simulink model "ES259A_BattVltgCorrln"  (R2013b)
settings: Solver=FixedStepDiscrete  SolverMode=SingleTasking  StartTime=0.0  StopTime=Inf  FixedStep=0.002  RelTol=1e-3
values from neighbouring files (symbols this model uses):
  BattVltgCorrlnAllwdVltgDif = DataDict.Calibration    [ES259A_BattVltgCorrln_DataDict.m]
  BattVltgCorrlnBattLoVltg = DataDict.Calibration    [ES259A_BattVltgCorrln_DataDict.m]
  BattVltgCorrlnBattOverVltg = DataDict.Calibration    [ES259A_BattVltgCorrln_DataDict.m]
  BattVltgCorrlnBattUnderVltg = DataDict.Calibration    [ES259A_BattVltgCorrln_DataDict.m]
  BattVltgCorrlnNtc0x03C0x0440x04CFailStep = DataDict.Calibration    [ES259A_BattVltgCorrln_DataDict.m]
  BattVltgCorrlnNtc0x03C0x0440x04CPassStep = DataDict.Calibration    [ES259A_BattVltgCorrln_DataDict.m]
  BattVltgCorrlnNtc0x03DFailStep = DataDict.Calibration    [ES259A_BattVltgCorrln_DataDict.m]
  BattVltgCorrlnNtc0x03DPassStep = DataDict.Calibration    [ES259A_BattVltgCorrln_DataDict.m]
  BattVltgCorrlnNtc0x0B0FailStep = DataDict.Calibration    [ES259A_BattVltgCorrln_DataDict.m]
  BattVltgCorrlnNtc0x0B0PassStep = DataDict.Calibration    [ES259A_BattVltgCorrln_DataDict.m]
  BattVltgCorrlnNtc0x0B1FailStep = DataDict.Calibration    [ES259A_BattVltgCorrln_DataDict.m]
  BattVltgCorrlnNtc0x0B1PassStep = DataDict.Calibration    [ES259A_BattVltgCorrln_DataDict.m]
  BattVltgCorrlnNtc0x0B5FailStep = DataDict.Calibration    [ES259A_BattVltgCorrln_DataDict.m]
  BattVltgCorrlnNtc0x0B5PassStep = DataDict.Calibration    [ES259A_BattVltgCorrln_DataDict.m]
  BattVltgCorrlnRcvrlBattLoVltg = DataDict.Calibration    [ES259A_BattVltgCorrln_DataDict.m]
  BattVltgCorrlnRcvrlBattOverVltg = DataDict.Calibration    [ES259A_BattVltgCorrln_DataDict.m]
  BattVltgCorrlnRcvrlBattUnderVltg = DataDict.Calibration    [ES259A_BattVltgCorrln_DataDict.m]
  BattVltgCorrlnSysMinVltg = DataDict.ImprtdCal    [ES250A_BattVltg_DataDict.m]    (also in ES259A_BattVltgCorrln_DataDict.m = DataDict.Calibration)
  BattVltgSwdMax = DataDict.Calibration    [ES250A_BattVltg_DataDict.m]
  ELECGLBPRM_STRTUPSTPWRDISCNCTBTESTCMPL_CNT_U08 = DataDict.Constant    [ES999A_ElecGlbPrm_DataDict.m]
  SYSVLTGFLTDUALIVTR_CNT_U08 = DataDict.Constant    [ES259A_BattVltgCorrln_DataDict.m]
undefined symbols (not defined in the file or in its folder): NtcNr1, NtcSts1, SigQlfr1
libraries: simulink x14
(part 3 of 7)

== system ES259A_BattVltgCorrln/BattVltgCorrln/BattVltgCorrlnPer1/Battery Voltage Diagnostics/Inhibition Off/BattVltg > OverVltg/SetNtcStsB0 ==
  note: Only pass values 2 or 3 as input to NtcSts.
      | 2: PrePassd
      | 3: PreFaild
  NtcNr : Inport
  NtcStInfo : Inport  Port=2
  NtcSts : Inport  Port=3
  DebStep : Inport  Port=4
  Copyright1 : Subsystem  Description=|  mask(Copyright Information){none=on}
      | Copyright info block.                                               
      |                                                                     
      | Place copyright information at the top of every subsystem in design.
      mask prompts: none "No parameters"
      mask help: Place copyright information at the top of every subsystem in design.
      mask Display:
      | NxtrConf = 'Nexteer Confidential';
      | 
      | sys = bdroot; %handle for the current model ("system")
      | first = get_param(sys,'Created');
      | if(isempty(first))
      |     first = datestr(now,'yyyy');
      | else
      |     first = first(end-3:end);  %year is last four digits
      | end
      | 
      | last = get_param(sys,'LastModifiedDate');
      | if isempty(last)
      |     last = datestr(now,'yyyy');
      | else
      |     last = last(end-3:end);
      | end
      | 
      | if strcmp(first,last)
      |     fprintf('%s\nCopyright  %s Nexteer',NxtrConf,first);
      | else
      |     fprintf('%s\n%s%s-%s Nexteer',NxtrConf,char(169),first,last);
      | end
  Data Store Write1 : DataStoreWrite  RequirementInfo={} %GIDa_a76b7c1b_e703_40d3_920b_5685c046c797  DataStoreName=NtcQlfr44
  ISO Fault Debounce Design NOT TO BE IMPLEMENTED IN THIS FDD USED ONLY FOR SIMULATION PURPOSES : Stateflow chart  TreatAsAtomicUnit=on
  Only here because I could not get model to run with enumerations in the stateflow diagram : DataTypeConversion  OutDataTypeStr=uint8
  Terminator : Terminator
  Terminator1 : Terminator
  wires:
  NtcStInfo/1 -> Terminator1/1
  NtcNr/1 -> Terminator/1
  NtcSts/1 -> Only here because I could not get model to run with enumerations in the stateflow diagram/1
  DebStep/1 -> ISO Fault Debounce Design NOT TO BE IMPLEMENTED IN THIS FDD USED ONLY FOR SIMULATION PURPOSES/2(DebStep)
  Only here because I could not get model to run with enumerations in the stateflow diagram/1 -> ISO Fault Debounce Design NOT TO BE IMPLEMENTED IN THIS FDD USED ONLY FOR SIMULATION PURPOSES/1(NtcSts)
  ISO Fault Debounce Design NOT TO BE IMPLEMENTED IN THIS FDD USED ONLY FOR SIMULATION PURPOSES/1(Qualifier) -> Data Store Write1/1

== system ES259A_BattVltgCorrln/BattVltgCorrln/BattVltgCorrlnPer1/Battery Voltage Diagnostics/Inhibition Off/BattVltg > OverVltg/SetNtcStsB1 ==
  note: Only pass values 2 or 3 as input to NtcSts.
      | 2: PrePassd
      | 3: PreFaild
  NtcNr : Inport
  NtcStInfo : Inport  Port=2
  NtcSts : Inport  Port=3
  DebStep : Inport  Port=4
  Copyright1 : Subsystem  Description=|  mask(Copyright Information){none=on}
      | Copyright info block.                                               
      |                                                                     
      | Place copyright information at the top of every subsystem in design.
      mask prompts: none "No parameters"
      mask help: Place copyright information at the top of every subsystem in design.
      mask Display:
      | NxtrConf = 'Nexteer Confidential';
      | 
      | sys = bdroot; %handle for the current model ("system")
      | first = get_param(sys,'Created');
      | if(isempty(first))
      |     first = datestr(now,'yyyy');
      | else
      |     first = first(end-3:end);  %year is last four digits
      | end
      | 
      | last = get_param(sys,'LastModifiedDate');
      | if isempty(last)
      |     last = datestr(now,'yyyy');
      | else
      |     last = last(end-3:end);
      | end
      | 
      | if strcmp(first,last)
      |     fprintf('%s\nCopyright  %s Nexteer',NxtrConf,first);
      | else
      |     fprintf('%s\n%s%s-%s Nexteer',NxtrConf,char(169),first,last);
      | end
  Data Store Write1 : DataStoreWrite  RequirementInfo={} %GIDa_e78ef1d1_c2fb_41bc_8318_ed3d0db9f38f  DataStoreName=NtcQlfr44
  ISO Fault Debounce Design NOT TO BE IMPLEMENTED IN THIS FDD USED ONLY FOR SIMULATION PURPOSES : Stateflow chart  TreatAsAtomicUnit=on
  Only here because I could not get model to run with enumerations in the stateflow diagram : DataTypeConversion  OutDataTypeStr=uint8
  Terminator : Terminator
  Terminator1 : Terminator
  wires:
  NtcStInfo/1 -> Terminator1/1
  NtcNr/1 -> Terminator/1
  NtcSts/1 -> Only here because I could not get model to run with enumerations in the stateflow diagram/1
  DebStep/1 -> ISO Fault Debounce Design NOT TO BE IMPLEMENTED IN THIS FDD USED ONLY FOR SIMULATION PURPOSES/2(DebStep)
  Only here because I could not get model to run with enumerations in the stateflow diagram/1 -> ISO Fault Debounce Design NOT TO BE IMPLEMENTED IN THIS FDD USED ONLY FOR SIMULATION PURPOSES/1(NtcSts)
  ISO Fault Debounce Design NOT TO BE IMPLEMENTED IN THIS FDD USED ONLY FOR SIMULATION PURPOSES/1(Qualifier) -> Data Store Write1/1

== system ES259A_BattVltgCorrln/BattVltgCorrln/BattVltgCorrlnPer1/Battery Voltage Diagnostics/Inhibition Off/BattVltg > OverVltg/SetNtcStsB5 ==
  note: Only pass values 2 or 3 as input to NtcSts.
      | 2: PrePassd
      | 3: PreFaild
  NtcNr : Inport
  NtcStInfo : Inport  Port=2
  NtcSts : Inport  Port=3
  DebStep : Inport  Port=4
  Copyright1 : Subsystem  Description=|  mask(Copyright Information){none=on}
      | Copyright info block.                                               
      |                                                                     
      | Place copyright information at the top of every subsystem in design.
      mask prompts: none "No parameters"
      mask help: Place copyright information at the top of every subsystem in design.
      mask Display:
      | NxtrConf = 'Nexteer Confidential';
      | 
      | sys = bdroot; %handle for the current model ("system")
      | first = get_param(sys,'Created');
      | if(isempty(first))
      |     first = datestr(now,'yyyy');
      | else
      |     first = first(end-3:end);  %year is last four digits
      | end
      | 
      | last = get_param(sys,'LastModifiedDate');
      | if isempty(last)
      |     last = datestr(now,'yyyy');
      | else
      |     last = last(end-3:end);
      | end
      | 
      | if strcmp(first,last)
      |     fprintf('%s\nCopyright  %s Nexteer',NxtrConf,first);
      | else
      |     fprintf('%s\n%s%s-%s Nexteer',NxtrConf,char(169),first,last);
      | end
  Data Store Write1 : DataStoreWrite  RequirementInfo={} %GIDa_85e34c1f_27cb_43cc_bc94_0eeb023d6696  DataStoreName=NtcQlfr44
  ISO Fault Debounce Design NOT TO BE IMPLEMENTED IN THIS FDD USED ONLY FOR SIMULATION PURPOSES : Stateflow chart  TreatAsAtomicUnit=on
  Only here because I could not get model to run with enumerations in the stateflow diagram : DataTypeConversion  OutDataTypeStr=uint8
  Terminator : Terminator
  Terminator1 : Terminator
  wires:
  NtcStInfo/1 -> Terminator1/1
  NtcNr/1 -> Terminator/1
  NtcSts/1 -> Only here because I could not get model to run with enumerations in the stateflow diagram/1
  DebStep/1 -> ISO Fault Debounce Design NOT TO BE IMPLEMENTED IN THIS FDD USED ONLY FOR SIMULATION PURPOSES/2(DebStep)
  Only here because I could not get model to run with enumerations in the stateflow diagram/1 -> ISO Fault Debounce Design NOT TO BE IMPLEMENTED IN THIS FDD USED ONLY FOR SIMULATION PURPOSES/1(NtcSts)
  ISO Fault Debounce Design NOT TO BE IMPLEMENTED IN THIS FDD USED ONLY FOR SIMULATION PURPOSES/1(Qualifier) -> Data Store Write1/1

== system ES259A_BattVltgCorrln/BattVltgCorrln/BattVltgCorrlnPer1/Battery Voltage Diagnostics/Inhibition Off/LowVltg <= Batt <= OverVltg/Copyright1 ==

== system ES259A_BattVltgCorrln/BattVltgCorrln/BattVltgCorrlnPer1/Battery Voltage Diagnostics/Inhibition Off/LowVltg <= Batt <= OverVltg/If Action ==
  Action Port : ActionPort  ActionType=then
  Copyright1 : Subsystem  Description=|  mask(Copyright Information){none=on}
      | Copyright info block.                                               
      |                                                                     
      | Place copyright information at the top of every subsystem in design.
      mask prompts: none "No parameters"
      mask help: Place copyright information at the top of every subsystem in design.
      mask Display:
      | NxtrConf = 'Nexteer Confidential';
      | 
      | sys = bdroot; %handle for the current model ("system")
      | first = get_param(sys,'Created');
      | if(isempty(first))
      |     first = datestr(now,'yyyy');
      | else
      |     first = first(end-3:end);  %year is last four digits
      | end
      | 
      | last = get_param(sys,'LastModifiedDate');
      | if isempty(last)
      |     last = datestr(now,'yyyy');
      | else
      |     last = last(end-3:end);
      | end
      | 
      | if strcmp(first,last)
      |     fprintf('%s\nCopyright  %s Nexteer',NxtrConf,first);
      | else
      |     fprintf('%s\n%s%s-%s Nexteer',NxtrConf,char(169),first,last);
      | end
  DebStep2 : Constant  RequirementInfo={} %GIDa_1195c223_b15e_4011_a962_e2535975fc54  Value=BattVltgCorrlnNtc0x0B0PassStep
  DebStep3 : Constant  RequirementInfo={} %GIDa_99fae57e_0058_4828_94a1_2dd84bab7ddd  Value=BattVltgCorrlnNtc0x0B5PassStep
  Ntc Number (0x0B0) : Constant  RequirementInfo={} %GIDa_6ab020f2_68ae_4d7d_802f_3e8133867873  Value=NtcNr1.NTCNR_0X0B0
  Ntc Number (0x0B5) : Constant  RequirementInfo={} %GIDa_a4324f28_b20d_402e_a309_2007428a63d6  Value=NtcNr1.NTCNR_0X0B5
  NtcStInfo : Constant  RequirementInfo={} %GIDa_1f4ecd0b_fa9a_40d4_99d0_dabff1a56be4  Value=0
  NtcStInfo2 : Constant  RequirementInfo={} %GIDa_eba6cb61_26f3_4ab3_b75b_6ddb400f4594  Value=0
  SetNtcStsB0 : Subsystem  RequirementInfo={} %GIDa_2a7d46a2_3af2_4810_a050_3f0802d49757
      settings: RTWSystemCode=Inline
  SetNtcStsB5 : Subsystem  RequirementInfo={} %GIDa_0fdd3e1d_711a_4556_b935_f47cfbb83207
      settings: RTWSystemCode=Inline
  Status Type1 : Constant  Value=NtcSts1.NTCSTS_PREPASSD
  Status Type4 : Constant  Value=NtcSts1.NTCSTS_PREPASSD
  wires:
  NtcStInfo/1 -> SetNtcStsB5/2(NtcStInfo)
  DebStep2/1 -> SetNtcStsB0/4(DebStep)
  Status Type1/1 -> SetNtcStsB0/3(NtcSts)
  NtcStInfo2/1 -> SetNtcStsB0/2(NtcStInfo)
  DebStep3/1 -> SetNtcStsB5/4(DebStep)
  Status Type4/1 -> SetNtcStsB5/3(NtcSts)
  Ntc Number (0x0B5)/1 -> SetNtcStsB5/1(NtcNr)
  Ntc Number (0x0B0)/1 -> SetNtcStsB0/1(NtcNr)

== system ES259A_BattVltgCorrln/BattVltgCorrln/BattVltgCorrlnPer1/Battery Voltage Diagnostics/Inhibition Off/LowVltg <= Batt <= OverVltg/If Action 1 ==
  Action Port : ActionPort  ActionType=elseif
  Copyright1 : Subsystem  Description=|  mask(Copyright Information){none=on}
      | Copyright info block.                                               
      |                                                                     
      | Place copyright information at the top of every subsystem in design.
      mask prompts: none "No parameters"
      mask help: Place copyright information at the top of every subsystem in design.
      mask Display:
      | NxtrConf = 'Nexteer Confidential';
      | 
      | sys = bdroot; %handle for the current model ("system")
      | first = get_param(sys,'Created');
      | if(isempty(first))
      |     first = datestr(now,'yyyy');
      | else
      |     first = first(end-3:end);  %year is last four digits
      | end
      | 
      | last = get_param(sys,'LastModifiedDate');
      | if isempty(last)
      |     last = datestr(now,'yyyy');
      | else
      |     last = last(end-3:end);
      | end
      | 
      | if strcmp(first,last)
      |     fprintf('%s\nCopyright  %s Nexteer',NxtrConf,first);
      | else
      |     fprintf('%s\n%s%s-%s Nexteer',NxtrConf,char(169),first,last);
      | end
  DebStep1 : Constant  RequirementInfo={} %GIDa_425365a2_390c_44cd_9124_5af2bf078374  Value=BattVltgCorrlnNtc0x0B1PassStep
  DebStep2 : Constant  RequirementInfo={} %GIDa_2051676b_ef0e_4e01_8698_05605269ab07  Value=BattVltgCorrlnNtc0x0B0PassStep
  Ntc Number (0x0B0) : Constant  RequirementInfo={} %GIDa_07c72315_2212_4b8a_a1bc_c51c72ee164e  Value=NtcNr1.NTCNR_0X0B0
  Ntc Number (0x0B1) : Constant  RequirementInfo={} %GIDa_683af33c_7867_4b16_9ead_17401dc3d862  Value=NtcNr1.NTCNR_0X0B1
  NtcStInfo1 : Constant  RequirementInfo={} %GIDa_0ba3a7e6_d64c_4d8a_bbae_943d01a71b70  Value=0
  NtcStInfo2 : Constant  RequirementInfo={} %GIDa_da72ece6_e4c5_468e_93c2_353b23db9d4f  Value=0
  SetNtcStsB0 : Subsystem  RequirementInfo={} %GIDa_66b34f22_d914_4cfb_ac31_be92138ce7ad
      settings: RTWSystemCode=Inline
  SetNtcStsB1 : Subsystem  RequirementInfo={} %GIDa_49b65210_4544_41bd_be96_fd2468f80b16
      settings: RTWSystemCode=Inline
  Status Type1 : Constant  Value=NtcSts1.NTCSTS_PREPASSD
  Status Type4 : Constant  Value=NtcSts1.NTCSTS_PREPASSD
  wires:
  Ntc Number (0x0B0)/1 -> SetNtcStsB0/1(NtcNr)
  Ntc Number (0x0B1)/1 -> SetNtcStsB1/1(NtcNr)
  NtcStInfo2/1 -> SetNtcStsB0/2(NtcStInfo)
  Status Type4/1 -> SetNtcStsB1/3(NtcSts)
  NtcStInfo1/1 -> SetNtcStsB1/2(NtcStInfo)
  Status Type1/1 -> SetNtcStsB0/3(NtcSts)
  DebStep2/1 -> SetNtcStsB0/4(DebStep)
  DebStep1/1 -> SetNtcStsB1/4(DebStep)

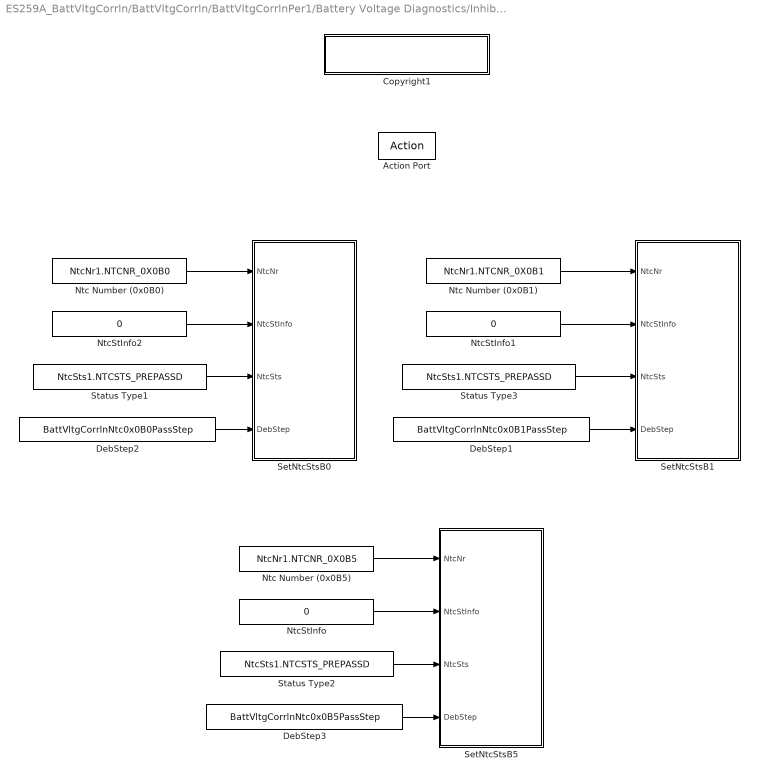
== system ES259A_BattVltgCorrln/BattVltgCorrln/BattVltgCorrlnPer1/Battery Voltage Diagnostics/Inhibition Off/LowVltg <= Batt <= OverVltg/No Fault Condition ==
  Action Port : ActionPort  ActionType=else
  Copyright1 : Subsystem  Description=|  mask(Copyright Information){none=on}
      | Copyright info block.                                               
      |                                                                     
      | Place copyright information at the top of every subsystem in design.
      mask prompts: none "No parameters"
      mask help: Place copyright information at the top of every subsystem in design.
      mask Display:
      | NxtrConf = 'Nexteer Confidential';
      | 
      | sys = bdroot; %handle for the current model ("system")
      | first = get_param(sys,'Created');
      | if(isempty(first))
      |     first = datestr(now,'yyyy');
      | else
      |     first = first(end-3:end);  %year is last four digits
      | end
      | 
      | last = get_param(sys,'LastModifiedDate');
      | if isempty(last)
      |     last = datestr(now,'yyyy');
      | else
      |     last = last(end-3:end);
      | end
      | 
      | if strcmp(first,last)
      |     fprintf('%s\nCopyright  %s Nexteer',NxtrConf,first);
      | else
      |     fprintf('%s\n%s%s-%s Nexteer',NxtrConf,char(169),first,last);
      | end
  DebStep1 : Constant  RequirementInfo={} %GIDa_45843794_75e7_46e2_ac75_531881001e0d  Value=BattVltgCorrlnNtc0x0B1PassStep
  DebStep2 : Constant  RequirementInfo={} %GIDa_346538d6_4570_4088_a4fe_c52f9190ad5f  Value=BattVltgCorrlnNtc0x0B0PassStep
  DebStep3 : Constant  RequirementInfo={} %GIDa_289d1d4e_b0db_4723_99d9_fb0d345f0978  Value=BattVltgCorrlnNtc0x0B5PassStep
  Ntc Number (0x0B0) : Constant  RequirementInfo={} %GIDa_50917ca9_6df5_4a8d_9e47_18831867c7d8  Value=NtcNr1.NTCNR_0X0B0
  Ntc Number (0x0B1) : Constant  RequirementInfo={} %GIDa_1fba47b3_01aa_4534_9e49_233f4459d2fd  Value=NtcNr1.NTCNR_0X0B1
  Ntc Number (0x0B5) : Constant  RequirementInfo={} %GIDa_ca04610d_bfb2_41e1_b1dd_f9a4358d4b4c  Value=NtcNr1.NTCNR_0X0B5
  NtcStInfo : Constant  RequirementInfo={} %GIDa_228080e4_fdde_4821_be2d_df0fca86c055  Value=0
  NtcStInfo1 : Constant  RequirementInfo={} %GIDa_20255a97_d6a6_45c6_8b9f_184349705374  Value=0
  NtcStInfo2 : Constant  RequirementInfo={} %GIDa_be0271cc_9791_4872_a529_2d201415ac9f  Value=0
  SetNtcStsB0 : Subsystem  RequirementInfo={} %GIDa_6e25ce43_eae7_436f_ab86_2efca104675b
      settings: RTWSystemCode=Inline
  SetNtcStsB1 : Subsystem  RequirementInfo={} %GIDa_beea754a_5fe2_46e4_87a4_8091c8202fe6
      settings: RTWSystemCode=Inline
  SetNtcStsB5 : Subsystem  RequirementInfo={} %GIDa_c5002f19_e7bb_4186_8404_81cfdd7a4744
      settings: RTWSystemCode=Inline
  Status Type1 : Constant  Value=NtcSts1.NTCSTS_PREPASSD
  Status Type2 : Constant  Value=NtcSts1.NTCSTS_PREPASSD
  Status Type3 : Constant  Value=NtcSts1.NTCSTS_PREPASSD
  wires:
  DebStep1/1 -> SetNtcStsB1/4(DebStep)
  NtcStInfo/1 -> SetNtcStsB5/2(NtcStInfo)
  DebStep2/1 -> SetNtcStsB0/4(DebStep)
  Status Type1/1 -> SetNtcStsB0/3(NtcSts)
  NtcStInfo1/1 -> SetNtcStsB1/2(NtcStInfo)
  Status Type3/1 -> SetNtcStsB1/3(NtcSts)
  NtcStInfo2/1 -> SetNtcStsB0/2(NtcStInfo)
  DebStep3/1 -> SetNtcStsB5/4(DebStep)
  Status Type2/1 -> SetNtcStsB5/3(NtcSts)
  Ntc Number (0x0B5)/1 -> SetNtcStsB5/1(NtcNr)
  Ntc Number (0x0B1)/1 -> SetNtcStsB1/1(NtcNr)
  Ntc Number (0x0B0)/1 -> SetNtcStsB0/1(NtcNr)

== system ES259A_BattVltgCorrln/BattVltgCorrln/BattVltgCorrlnPer1/Battery Voltage Diagnostics/Inhibition Off/UnderVltg <= BattVltg < LowVltg/Copyright1 ==

== system ES259A_BattVltgCorrln/BattVltgCorrln/BattVltgCorrlnPer1/Battery Voltage Diagnostics/Inhibition Off/UnderVltg <= BattVltg < LowVltg/If Action ==
  Action Port : ActionPort  ActionType=then
  Copyright1 : Subsystem  Description=|  mask(Copyright Information){none=on}
      | Copyright info block.                                               
      |                                                                     
      | Place copyright information at the top of every subsystem in design.
      mask prompts: none "No parameters"
      mask help: Place copyright information at the top of every subsystem in design.
      mask Display:
      | NxtrConf = 'Nexteer Confidential';
      | 
      | sys = bdroot; %handle for the current model ("system")
      | first = get_param(sys,'Created');
      | if(isempty(first))
      |     first = datestr(now,'yyyy');
      | else
      |     first = first(end-3:end);  %year is last four digits
      | end
      | 
      | last = get_param(sys,'LastModifiedDate');
      | if isempty(last)
      |     last = datestr(now,'yyyy');
      | else
      |     last = last(end-3:end);
      | end
      | 
      | if strcmp(first,last)
      |     fprintf('%s\nCopyright  %s Nexteer',NxtrConf,first);
      | else
      |     fprintf('%s\n%s%s-%s Nexteer',NxtrConf,char(169),first,last);
      | end
  DebStep1 : Constant  RequirementInfo={} %GIDa_363579d4_bd35_4b95_93e8_e62681a8443d  Value=BattVltgCorrlnNtc0x0B5PassStep
  DebStep2 : Constant  RequirementInfo={} %GIDa_6d1efd6a_7626_451f_8de6_d6ebe86bd348  Value=BattVltgCorrlnNtc0x0B1FailStep
  Ntc Number (0x0B1) : Constant  RequirementInfo={} %GIDa_b3c9ba86_e2ed_4870_a73a_5765450e312b  Value=NtcNr1.NTCNR_0X0B1
  Ntc Number (0x0B5) : Constant  RequirementInfo={} %GIDa_2c24a252_7b55_4e6c_8c8e_129e3eb37823  Value=NtcNr1.NTCNR_0X0B5
  NtcStInfo : Constant  RequirementInfo={} %GIDa_d0c87613_0a28_4b16_9511_44879192ff30  Value=0
  NtcStInfo1 : Constant  RequirementInfo={} %GIDa_bdbd0a3b_eb95_43ed_9a08_6277ae4f65ad
  SetNtcStsB1 : Subsystem  RequirementInfo={} %GIDa_97ee16e6_892d_49b5_a507_34e34be0ce4e
      settings: RTWSystemCode=Inline
  SetNtcStsB5 : Subsystem  RequirementInfo={} %GIDa_fce64b9c_68f8_4e6c_9569_2ca30be4b0c0
      settings: RTWSystemCode=Inline
  Status Type3 : Constant  Value=NtcSts1.NTCSTS_PREFAILD
  Status Type4 : Constant  Value=NtcSts1.NTCSTS_PREPASSD
  wires:
  DebStep2/1 -> SetNtcStsB1/4(DebStep)
  NtcStInfo/1 -> SetNtcStsB5/2(NtcStInfo)
  NtcStInfo1/1 -> SetNtcStsB1/2(NtcStInfo)
  Status Type3/1 -> SetNtcStsB1/3(NtcSts)
  DebStep1/1 -> SetNtcStsB5/4(DebStep)
  Status Type4/1 -> SetNtcStsB5/3(NtcSts)
  Ntc Number (0x0B5)/1 -> SetNtcStsB5/1(NtcNr)
  Ntc Number (0x0B1)/1 -> SetNtcStsB1/1(NtcNr)

== system ES259A_BattVltgCorrln/BattVltgCorrln/BattVltgCorrlnPer1/Battery Voltage Diagnostics/Inhibition Off/UnderVltg <= BattVltg < LowVltg/If Action 1 ==
  Action Port : ActionPort  ActionType=else
  Copyright1 : Subsystem  Description=|  mask(Copyright Information){none=on}
      | Copyright info block.                                               
      |                                                                     
      | Place copyright information at the top of every subsystem in design.
      mask prompts: none "No parameters"
      mask help: Place copyright information at the top of every subsystem in design.
      mask Display:
      | NxtrConf = 'Nexteer Confidential';
      | 
      | sys = bdroot; %handle for the current model ("system")
      | first = get_param(sys,'Created');
      | if(isempty(first))
      |     first = datestr(now,'yyyy');
      | else
      |     first = first(end-3:end);  %year is last four digits
      | end
      | 
      | last = get_param(sys,'LastModifiedDate');
      | if isempty(last)
      |     last = datestr(now,'yyyy');
      | else
      |     last = last(end-3:end);
      | end
      | 
      | if strcmp(first,last)
      |     fprintf('%s\nCopyright  %s Nexteer',NxtrConf,first);
      | else
      |     fprintf('%s\n%s%s-%s Nexteer',NxtrConf,char(169),first,last);
      | end
  DebStep1 : Constant  RequirementInfo={} %GIDa_1d756443_8494_4603_8240_a0e56e46942a  Value=BattVltgCorrlnNtc0x0B1FailStep
  DebStep2 : Constant  RequirementInfo={} %GIDa_d7ac8eb1_c935_4eda_a3ce_f3a139372a27  Value=BattVltgCorrlnNtc0x0B0PassStep
  DebStep3 : Constant  RequirementInfo={} %GIDa_fa95d256_37e3_4b02_9b67_5b5a5a5551d5  Value=BattVltgCorrlnNtc0x0B5PassStep
  Ntc Number (0x0B0) : Constant  RequirementInfo={} %GIDa_aa653830_06df_43fc_9978_463d01747d56  Value=NtcNr1.NTCNR_0X0B0
  Ntc Number (0x0B1) : Constant  RequirementInfo={} %GIDa_1ad25427_f5ca_4563_9370_445148180997  Value=NtcNr1.NTCNR_0X0B1
  Ntc Number (0x0B5) : Constant  RequirementInfo={} %GIDa_2c305410_6eba_4bf9_b51a_c3013e20ffdb  Value=NtcNr1.NTCNR_0X0B5
  NtcStInfo : Constant  RequirementInfo={} %GIDa_c1879ab7_ce89_4f5a_99ac_47fb04737930  Value=0
  NtcStInfo1 : Constant  RequirementInfo={} %GIDa_8f405b15_ced1_406f_9cb9_fbab56c1facc
  NtcStInfo2 : Constant  RequirementInfo={} %GIDa_70d46ad7_2465_44d1_948b_adc35e714326  Value=0
  SetNtcStsB0 : Subsystem  RequirementInfo={} %GIDa_e3d97823_6b4e_4203_9dd5_937b02f0bd86
      settings: RTWSystemCode=Inline
  SetNtcStsB1 : Subsystem  RequirementInfo={} %GIDa_6d47a2b0_7370_4b84_b9de_20113ec31e43
      settings: RTWSystemCode=Inline
  SetNtcStsB5 : Subsystem  RequirementInfo={} %GIDa_8e33babd_4b89_48c8_8d77_69e579954146
      settings: RTWSystemCode=Inline
  Status Type1 : Constant  Value=NtcSts1.NTCSTS_PREPASSD
  Status Type3 : Constant  Value=NtcSts1.NTCSTS_PREFAILD
  Status Type4 : Constant  Value=NtcSts1.NTCSTS_PREPASSD
  wires:
  Ntc Number (0x0B0)/1 -> SetNtcStsB0/1(NtcNr)
  Ntc Number (0x0B1)/1 -> SetNtcStsB1/1(NtcNr)
  Ntc Number (0x0B5)/1 -> SetNtcStsB5/1(NtcNr)
  Status Type4/1 -> SetNtcStsB5/3(NtcSts)
  DebStep3/1 -> SetNtcStsB5/4(DebStep)
  NtcStInfo2/1 -> SetNtcStsB0/2(NtcStInfo)
  Status Type3/1 -> SetNtcStsB1/3(NtcSts)
  NtcStInfo1/1 -> SetNtcStsB1/2(NtcStInfo)
  Status Type1/1 -> SetNtcStsB0/3(NtcSts)
  DebStep2/1 -> SetNtcStsB0/4(DebStep)
  NtcStInfo/1 -> SetNtcStsB5/2(NtcStInfo)
  DebStep1/1 -> SetNtcStsB1/4(DebStep)

== system ES259A_BattVltgCorrln/BattVltgCorrln/BattVltgCorrlnPer1/WarmInit or Enable/Determine Correlation Status/Use Arbitraiton Voltage/Copyright1 ==

== system ES259A_BattVltgCorrln/BattVltgCorrln/BattVltgCorrlnPer1/WarmInit or Enable/Determine Correlation Status/Use Default Voltage/Copyright1 ==

== system ES259A_BattVltgCorrln/BattVltgCorrln/BattVltgCorrlnPer1/WarmInit or Enable/Determine Independent Signals/BattVltg Failed/Copyright1 ==

== system ES259A_BattVltgCorrln/BattVltgCorrln/BattVltgCorrlnPer1/WarmInit or Enable/Determine Independent Signals/BattVltg Passed/Copyright1 ==

== system ES259A_BattVltgCorrln/BattVltgCorrln/BattVltgCorrlnPer1/WarmInit or Enable/Determine Independent Signals/BattVltgSwd1 Failed/Copyright1 ==

== system ES259A_BattVltgCorrln/BattVltgCorrln/BattVltgCorrlnPer1/WarmInit or Enable/Determine Independent Signals/BattVltgSwd1 Passed/Copyright1 ==

== system ES259A_BattVltgCorrln/BattVltgCorrln/BattVltgCorrlnPer1/WarmInit or Enable/Determine Independent Signals/BattVltgSwd2 Failed/Copyright1 ==

== system ES259A_BattVltgCorrln/BattVltgCorrln/BattVltgCorrlnPer1/WarmInit or Enable/Determine Independent Signals/BattVltgSwd2 Passed/Copyright1 ==

== system ES259A_BattVltgCorrln/BattVltgCorrln/BattVltgCorrlnPer1/WarmInit or Enable/Determine Independent Signals/Diagnose Inputs/Copyright1 ==

== system ES259A_BattVltgCorrln/BattVltgCorrln/BattVltgCorrlnPer1/WarmInit or Enable/Determine Independent Signals/Diagnose Inputs/NTC 3C ==
  BattVltgOk : Inport
  Copyright1 : Subsystem  Description=|  mask(Copyright Information){none=on}
      | Copyright info block.                                               
      |                                                                     
      | Place copyright information at the top of every subsystem in design.
      mask prompts: none "No parameters"
      mask help: Place copyright information at the top of every subsystem in design.
      mask Display:
      | NxtrConf = 'Nexteer Confidential';
      | 
      | sys = bdroot; %handle for the current model ("system")
      | first = get_param(sys,'Created');
      | if(isempty(first))
      |     first = datestr(now,'yyyy');
      | else
      |     first = first(end-3:end);  %year is last four digits
      | end
      | 
      | last = get_param(sys,'LastModifiedDate');
      | if isempty(last)
      |     last = datestr(now,'yyyy');
      | else
      |     last = last(end-3:end);
      | end
      | 
      | if strcmp(first,last)
      |     fprintf('%s\nCopyright  %s Nexteer',NxtrConf,first);
      | else
      |     fprintf('%s\n%s%s-%s Nexteer',NxtrConf,char(169),first,last);
      | end
  "GetNtcQlfrSts " : Subsystem  RequirementInfo={} %GIDa_9e252bde_db44_433a_9c3e_c5c0da10312c  Priority=2
  NTC 0x03C : Constant  RequirementInfo={} %GIDa_cc25a7a0_0484_4f73_8186_a98240e9737c  Value=NtcNr1.NTCNR_0X03C  OutDataTypeStr=Enum: NtcNr1
  Return3 : Terminator
      settings: RequirementInfo={} %GIDa_f9a85be1_2888_4a9b_824f_2aa300759879
  SetNtcSts 0x03C : Subsystem  RequirementInfo="{'linktype_rmi_doors' '0000cf46 (/ESG Group/FDD Module Requirements/EA4 Specific/ES259A_BattVltgCorrln)' '#ES259A_126' 'true' 'REQ:  ES259A_126' '' ; 'linktype_rmi_doors' '0000cf46 (/ESG Group/FDD Module Requirements/EA4 Specific/ES259A_BattVltgCorrln)' '#ES259A_128' 'true' 'REQ:  ES259A_128' '' ; 'linktype_rmi_doors' '0000cf46 (/ESG Group/FDD Module Requirements/EA4 Specific/ES259A_BattVltgCorrln)' '#ES259A_148' 'true' 'REQ:  ES259A_148' '' ; 'linktype_rmi_doors' '0000cf46 (/ESG Group/FDD Module Requirements/EA4 Specific/ES259A_BattVltgCorrln)' '#ES259A_133' 'true' 'REQ:  ES259A_133' '' ; 'linktype_rmi_doors' '0000cf46 (/ESG Group/FDD Module Requirements/EA4 Specific/ES259A_BattVltgCorrln)' '#ES259A_132' 'true' 'REQ:  ES259A_132' '' } %GIDa_2b41bcc0_d4a3_40a2_92b1_6a70e9430527"  Priority=1
  Ntc0x03CQlfrSts : Outport
  wires:
  "GetNtcQlfrSts "/2(Ntc0x03CQlfrSts) -> Ntc0x03CQlfrSts/1
  NTC 0x03C/1 -> "GetNtcQlfrSts "/1(NtcNr)
  BattVltgOk/1 -> SetNtcSts 0x03C/1(BattVltgOk)
  "GetNtcQlfrSts "/1(Return) -> Return3/1

== system ES259A_BattVltgCorrln/BattVltgCorrln/BattVltgCorrlnPer1/WarmInit or Enable/Determine Independent Signals/Diagnose Inputs/NTC 3D ==
  BattVltgOk : Inport
  BattVltgSwd1Ok : Inport  Port=2
  BattVltgSwd2Ok : Inport  Port=3
  Add : Sum  Inputs=+++
  Copyright1 : Subsystem  Description=|  mask(Copyright Information){none=on}
      | Copyright info block.                                               
      |                                                                     
      | Place copyright information at the top of every subsystem in design.
      mask prompts: none "No parameters"
      mask help: Place copyright information at the top of every subsystem in design.
      mask Display:
      | NxtrConf = 'Nexteer Confidential';
      | 
      | sys = bdroot; %handle for the current model ("system")
      | first = get_param(sys,'Created');
      | if(isempty(first))
      |     first = datestr(now,'yyyy');
      | else
      |     first = first(end-3:end);  %year is last four digits
      | end
      | 
      | last = get_param(sys,'LastModifiedDate');
      | if isempty(last)
      |     last = datestr(now,'yyyy');
      | else
      |     last = last(end-3:end);
      | end
      | 
      | if strcmp(first,last)
      |     fprintf('%s\nCopyright  %s Nexteer',NxtrConf,first);
      | else
      |     fprintf('%s\n%s%s-%s Nexteer',NxtrConf,char(169),first,last);
      | end
  Data Store Write3 : DataStoreWrite  DataStoreName=dBattVltgCorrlnNtc0x03DQlfrSts
  Fail NTC 3D : Subsystem  TreatAsAtomicUnit=on
  GetNtcQlfrSts : Subsystem  RequirementInfo={} %GIDa_a8274c61_6604_48f4_a914_7410b0ebb962  Priority=2
  If : If  IfExpression=u1 <= 1
  NTC 0x03D : Constant  RequirementInfo={} %GIDa_01de9a88_a0d4_4b07_9d68_3f8d6819482a  Value=NtcNr1.NTCNR_0X03D  OutDataTypeStr=Enum: NtcNr1
  Pass NTC 3D : Subsystem
  Return3 : Terminator
      settings: RequirementInfo={} %GIDa_f8792081_4daa_47e3_9ef8_f4aa69609aa3
  wires:
  BattVltgOk/1 -> Add/1
  BattVltgSwd1Ok/1 -> Add/2
  BattVltgSwd2Ok/1 -> Add/3
  Add/1 -> If/1
  If/2 -> Pass NTC 3D/Action
  If/1 -> Fail NTC 3D/Action
  GetNtcQlfrSts/2(Ntc0x03DQlfrSts) -> Data Store Write3/1
  NTC 0x03D/1 -> GetNtcQlfrSts/1(NtcNr)
  GetNtcQlfrSts/1(Return) -> Return3/1

== system ES259A_BattVltgCorrln/BattVltgCorrln/BattVltgCorrlnPer1/WarmInit or Enable/Determine Independent Signals/Diagnose Inputs/NTC 44 ==
  BattVltgSwd1Ok : Inport
  DiagcStsIvtr1Inactv : Inport  Port=2
  Copyright1 : Subsystem  Description=|  mask(Copyright Information){none=on}
      | Copyright info block.                                               
      |                                                                     
      | Place copyright information at the top of every subsystem in design.
      mask prompts: none "No parameters"
      mask help: Place copyright information at the top of every subsystem in design.
      mask Display:
      | NxtrConf = 'Nexteer Confidential';
      | 
      | sys = bdroot; %handle for the current model ("system")
      | first = get_param(sys,'Created');
      | if(isempty(first))
      |     first = datestr(now,'yyyy');
      | else
      |     first = first(end-3:end);  %year is last four digits
      | end
      | 
      | last = get_param(sys,'LastModifiedDate');
      | if isempty(last)
      |     last = datestr(now,'yyyy');
      | else
      |     last = last(end-3:end);
      | end
      | 
      | if strcmp(first,last)
      |     fprintf('%s\nCopyright  %s Nexteer',NxtrConf,first);
      | else
      |     fprintf('%s\n%s%s-%s Nexteer',NxtrConf,char(169),first,last);
      | end
  GetNtcQlfrSts 0x044 : Subsystem  RequirementInfo={} %GIDa_86ede665_595b_4823_84be_4a11914ae3ac  Priority=3
  SetNtcSts 0x044 : Subsystem  RequirementInfo="{'linktype_rmi_doors' '0000cf46 (/ESG Group/FDD Module Requirements/EA4 Specific/ES259A_BattVltgCorrln)' '#ES259A_22' 'true' 'REQ:  ES259A_22' '' ; 'linktype_rmi_doors' '0000cf46 (/ESG Group/FDD Module Requirements/EA4 Specific/ES259A_BattVltgCorrln)' '#ES259A_25' 'true' 'REQ:  ES259A_25' '' ; 'linktype_rmi_doors' '0000cf46 (/ESG Group/FDD Module Requirements/EA4 Specific/ES259A_BattVltgCorrln)' '#ES259A_146' 'true' 'REQ:  ES259A_146' '' ; 'linktype_rmi_doors' '0000cf46 (/ESG Group/FDD Module Requirements/EA4 Specific/ES259A_BattVltgCorrln)' '#ES259A_142' 'true' 'REQ:  ES259A_142' '' ; 'linktype_rmi_doors' '0000cf46 (/ESG Group/FDD Module Requirements/EA4 Specific/ES259A_BattVltgCorrln)' '#ES259A_28' 'true' 'REQ:  ES259A_28' '' ; 'linktype_rmi_doors' '0000cf46 (/ESG Group/FDD Module Requirements/EA4 Specific/ES259A_BattVltgCorrln)' '#ES259A_31' 'true' 'REQ:  ES259A_31' '' } %GIDa_4b1756ca_45c5_49b1_8e87_1423b5b533a2"  Priority=1
  Ntc0x044QlfrSts : Outport  OutDataTypeStr=uint8
  wires:
  DiagcStsIvtr1Inactv/1 -> GetNtcQlfrSts 0x044/1(DiagcStsIvtr1Inactv), SetNtcSts 0x044/2(DiagcStsIvtr1Inactv)
  GetNtcQlfrSts 0x044/1(Ntc0x044QlfrSts) -> Ntc0x044QlfrSts/1
  BattVltgSwd1Ok/1 -> SetNtcSts 0x044/1(BattVltgSwd1Ok)

== system ES259A_BattVltgCorrln/BattVltgCorrln/BattVltgCorrlnPer1/WarmInit or Enable/Determine Independent Signals/Diagnose Inputs/NTC 4C ==
  BattVltgSwd2Ok : Inport
  DiagcStsIvtr2Inactv : Inport  Port=2
  Copyright1 : Subsystem  Description=|  mask(Copyright Information){none=on}
      | Copyright info block.                                               
      |                                                                     
      | Place copyright information at the top of every subsystem in design.
      mask prompts: none "No parameters"
      mask help: Place copyright information at the top of every subsystem in design.
      mask Display:
      | NxtrConf = 'Nexteer Confidential';
      | 
      | sys = bdroot; %handle for the current model ("system")
      | first = get_param(sys,'Created');
      | if(isempty(first))
      |     first = datestr(now,'yyyy');
      | else
      |     first = first(end-3:end);  %year is last four digits
      | end
      | 
      | last = get_param(sys,'LastModifiedDate');
      | if isempty(last)
      |     last = datestr(now,'yyyy');
      | else
      |     last = last(end-3:end);
      | end
      | 
      | if strcmp(first,last)
      |     fprintf('%s\nCopyright  %s Nexteer',NxtrConf,first);
      | else
      |     fprintf('%s\n%s%s-%s Nexteer',NxtrConf,char(169),first,last);
      | end
  GetNtcQlfrSts 0x04C : Subsystem  Priority=4
  SetNtcSts 0x04C : Subsystem  RequirementInfo="{'linktype_rmi_doors' '0000cf46 (/ESG Group/FDD Module Requirements/EA4 Specific/ES259A_BattVltgCorrln)' '#ES259A_87' 'true' 'REQ:  ES259A_87' '' ; 'linktype_rmi_doors' '0000cf46 (/ESG Group/FDD Module Requirements/EA4 Specific/ES259A_BattVltgCorrln)' '#ES259A_89' 'true' 'REQ:  ES259A_89' '' ; 'linktype_rmi_doors' '0000cf46 (/ESG Group/FDD Module Requirements/EA4 Specific/ES259A_BattVltgCorrln)' '#ES259A_147' 'true' 'REQ:  ES259A_147' '' ; 'linktype_rmi_doors' '0000cf46 (/ESG Group/FDD Module Requirements/EA4 Specific/ES259A_BattVltgCorrln)' '#ES259A_143' 'true' 'REQ:  ES259A_143' '' ; 'linktype_rmi_doors' '0000cf46 (/ESG Group/FDD Module Requirements/EA4 Specific/ES259A_BattVltgCorrln)' '#ES259A_91' 'true' 'REQ:  ES259A_91' '' ; 'linktype_rmi_doors' '0000cf46 (/ESG Group/FDD Module Requirements/EA4 Specific/ES259A_BattVltgCorrln)' '#ES259A_94' 'true' 'REQ:  ES259A_94' '' } %GIDa_f19b1705_d7bb_4587_b722_9efd4bee9804"  Priority=2
  Ntc0x04CQlfrSts : Outport
  wires:
  BattVltgSwd2Ok/1 -> SetNtcSts 0x04C/1(BattVltgSwd2Ok)
  GetNtcQlfrSts 0x04C/1(Ntc0x04CQlfrSts) -> Ntc0x04CQlfrSts/1
  DiagcStsIvtr2Inactv/1 -> SetNtcSts 0x04C/2(DiagcStsIvtr2Inactv), GetNtcQlfrSts 0x04C/1(DiagcStsIvtr2Inactv)

== system ES259A_BattVltgCorrln/BattVltgCorrln/BattVltgCorrlnPer1/WarmInit or Enable/Determine Independent Signals/Use Arbitraiton Voltage/Copyright1 ==

== system ES259A_BattVltgCorrln/BattVltgCorrln/BattVltgCorrlnPer1/WarmInit or Enable/Determine Independent Signals/Use Default Voltage/Copyright1 ==

== system ES259A_BattVltgCorrln/BattVltgCorrln/BattVltgCorrlnPer1/WarmInit or Enable/Instantaneous Correlation/Correlation Check/BattVltg vs BattVltgSwd1 ==
  BattVltg : Inport  RequirementInfo={} %GIDa_e5a1e11a_ed2d_424a_97f6_18945350ad81
  BattVltgSwd1 : Inport  RequirementInfo={} %GIDa_6f5ec9fa_bfea_4be4_ad6b_ec4e11dfc24f  Port=2
  BattVltgCorrlnAllwdVltgDif : Inport  RequirementInfo={} %GIDa_33b9ab93_db2d_42a3_bbdf_270fc3168584  Port=3
  BattVltg <= 16 : Subsystem  TreatAsAtomicUnit=on
  BattVltg > 16 : Subsystem  TreatAsAtomicUnit=on
  Copyright1 : Subsystem  Description=|  RequirementInfo={} %GIDa_9bd21408_dc44_4581_bdee_9392e9b4fdaa  mask(Copyright Information){none=on}
      | Copyright info block.                                               
      |                                                                     
      | Place copyright information at the top of every subsystem in design.
      mask prompts: none "No parameters"
      mask help: Place copyright information at the top of every subsystem in design.
      mask Display:
      | NxtrConf = 'Nexteer Confidential';
      | 
      | sys = bdroot; %handle for the current model ("system")
      | first = get_param(sys,'Created');
      | if(isempty(first))
      |     first = datestr(now,'yyyy');
      | else
      |     first = first(end-3:end);  %year is last four digits
      | end
      | 
      | last = get_param(sys,'LastModifiedDate');
      | if isempty(last)
      |     last = datestr(now,'yyyy');
      | else
      |     last = last(end-3:end);
      | end
      | 
      | if strcmp(first,last)
      |     fprintf('%s\nCopyright  %s Nexteer',NxtrConf,first);
      | else
      |     fprintf('%s\n%s%s-%s Nexteer',NxtrConf,char(169),first,last);
      | end
  If : If  NumInputs=2  IfExpression=u1 <= u2
  Maximum Switched Voltage : Constant  Value=BattVltgSwdMax
  Merge : Merge
  TestOk_Lgc : Outport  RequirementInfo={} %GIDa_6c1e348a_2378_4b4d_8767_c56e8bfb4f6e
  wires:
  BattVltgCorrlnAllwdVltgDif/1 -> BattVltg <= 16/3(BattVltgCorrlnAllwdVltgDif), BattVltg > 16/2(BattVltgCorrlnAllwdVltgDif)
  BattVltg > 16/1(TestOk_Lgc) -> Merge/2
  BattVltg <= 16/1(TestOk_Lgc) -> Merge/1
  Merge/1 -> TestOk_Lgc/1
  Maximum Switched Voltage/1 -> If/2
  BattVltgSwd1/1 -> BattVltg <= 16/2(BattVltgSwd1), BattVltg > 16/1(BattVltgSwd1)
  BattVltg/1 -> BattVltg <= 16/1(BattVltg), If/1
  If/2 -> BattVltg > 16/Action
  If/1 -> BattVltg <= 16/Action

== system ES259A_BattVltgCorrln/BattVltgCorrln/BattVltgCorrlnPer1/WarmInit or Enable/Instantaneous Correlation/Correlation Check/BattVltgSwd1 vs BattVltgSwd2 ==
  BattVltgSwd1 : Inport  RequirementInfo={} %GIDa_89bee9d6_6651_4b36_8dbf_31848cef7f42
  BattVltgSwd2 : Inport  RequirementInfo={} %GIDa_dacc81d8_cdfc_480a_926d_932a76437c32  Port=2
  BattVltgCorrlnAllwdVltgDif : Inport  RequirementInfo={} %GIDa_38466d1c_9b7d_4008_b7ec_039bcba48116  Port=3
  Abs2 : Abs  RequirementInfo={} %GIDa_1fcfb709_7c95_4b0e_8330_cfa52db9132c  OutDataTypeStr=single
  Add : Sum
  Add1 : Sum  RequirementInfo={} %GIDa_928b074a_0d8b_43b1_bf49_3ac2082085c4  Inputs=+-  AccumDataTypeStr=single
  Copyright1 : Subsystem  Description=|  RequirementInfo={} %GIDa_0403d705_46b3_4dc6_8fa8_2545412691a4  mask(Copyright Information){none=on}
      | Copyright info block.                                               
      |                                                                     
      | Place copyright information at the top of every subsystem in design.
      mask prompts: none "No parameters"
      mask help: Place copyright information at the top of every subsystem in design.
      mask Display:
      | NxtrConf = 'Nexteer Confidential';
      | 
      | sys = bdroot; %handle for the current model ("system")
      | first = get_param(sys,'Created');
      | if(isempty(first))
      |     first = datestr(now,'yyyy');
      | else
      |     first = first(end-3:end);  %year is last four digits
      | end
      | 
      | last = get_param(sys,'LastModifiedDate');
      | if isempty(last)
      |     last = datestr(now,'yyyy');
      | else
      |     last = last(end-3:end);
      | end
      | 
      | if strcmp(first,last)
      |     fprintf('%s\nCopyright  %s Nexteer',NxtrConf,first);
      | else
      |     fprintf('%s\n%s%s-%s Nexteer',NxtrConf,char(169),first,last);
      | end
  Logical Operator : Logic  Inputs=3  AllPortsSameDT=off  OutDataTypeStr=boolean
  Maximum Switched Voltage : Constant  Value=BattVltgSwdMax
  Relational Operator : RelationalOperator  RequirementInfo={} %GIDa_734b622e_3b63_447c_b060_0ea29f514172  Operator=<=  OutDataTypeStr=boolean
  Relational Operator1 : RelationalOperator  RequirementInfo={} %GIDa_c7cefba9_ebab_4aab_b6d0_108cf118f9af  Operator=<=  OutDataTypeStr=boolean
  Relational Operator2 : RelationalOperator  RequirementInfo={} %GIDa_37c16149_0837_40d2_bb08_a52aeb2d1584  Operator=<=  OutDataTypeStr=boolean
  TestOk_Lgc : Outport  RequirementInfo={} %GIDa_c0117c80_be69_4099_b449_eeb7f8cab207
  wires:
  Relational Operator1/1 -> Logical Operator/2
  Add/1 -> Relational Operator1/2, Relational Operator2/2
  BattVltgCorrlnAllwdVltgDif/1 -> Relational Operator/2, Add/1
  Add1/1 -> Abs2/1
  Relational Operator/1 -> Logical Operator/1
  Relational Operator2/1 -> Logical Operator/3
  Logical Operator/1 -> TestOk_Lgc/1
  Maximum Switched Voltage/1 -> Add/2
  BattVltgSwd1/1 -> Add1/1, Relational Operator1/1
  BattVltgSwd2/1 -> Add1/2, Relational Operator2/1
  Abs2/1 -> Relational Operator/1

== system ES259A_BattVltgCorrln/BattVltgCorrln/BattVltgCorrlnPer1/WarmInit or Enable/Instantaneous Correlation/Correlation Check/BattVltgSwd2 vs BattVltg ==
  BattVltg : Inport  RequirementInfo={} %GIDa_4b9c33a3_6b2e_4993_a7c0_909a2fb795fe
  BattVltgSwd2 : Inport  RequirementInfo={} %GIDa_265a205f_68b1_4551_8f85_d1703e94914c  Port=2
  BattVltgCorrlnAllwdVltgDif : Inport  RequirementInfo={} %GIDa_eb3f4a04_3000_48f1_a9b0_a099e4471648  Port=3
  BattVltg <= 16 : Subsystem  TreatAsAtomicUnit=on
  BattVltg > 16 : Subsystem  TreatAsAtomicUnit=on
  Copyright1 : Subsystem  Description=|  RequirementInfo={} %GIDa_1bd1db2c_1c71_48ae_8b74_c309faa62218  mask(Copyright Information){none=on}
      | Copyright info block.                                               
      |                                                                     
      | Place copyright information at the top of every subsystem in design.
      mask prompts: none "No parameters"
      mask help: Place copyright information at the top of every subsystem in design.
      mask Display:
      | NxtrConf = 'Nexteer Confidential';
      | 
      | sys = bdroot; %handle for the current model ("system")
      | first = get_param(sys,'Created');
      | if(isempty(first))
      |     first = datestr(now,'yyyy');
      | else
      |     first = first(end-3:end);  %year is last four digits
      | end
      | 
      | last = get_param(sys,'LastModifiedDate');
      | if isempty(last)
      |     last = datestr(now,'yyyy');
      | else
      |     last = last(end-3:end);
      | end
      | 
      | if strcmp(first,last)
      |     fprintf('%s\nCopyright  %s Nexteer',NxtrConf,first);
      | else
      |     fprintf('%s\n%s%s-%s Nexteer',NxtrConf,char(169),first,last);
      | end
  If : If  NumInputs=2  IfExpression=u1 <= u2
  Maximum Switched Voltage : Constant  Value=BattVltgSwdMax
  Merge : Merge
  TestOk_Lgc : Outport  RequirementInfo={} %GIDa_5889f0ad_6b00_4902_b33d_d2cef3c15d7b
  wires:
  BattVltg > 16/1(TestOk_Lgc) -> Merge/2
  BattVltg <= 16/1(TestOk_Lgc) -> Merge/1
  Merge/1 -> TestOk_Lgc/1
  Maximum Switched Voltage/1 -> If/2
  BattVltgCorrlnAllwdVltgDif/1 -> BattVltg <= 16/3("BattVltgCorrlnAllwdVltgDif "), BattVltg > 16/2(BattVltgCorrlnAllwdVltgDif)
  BattVltgSwd2/1 -> BattVltg <= 16/2(BattVltgSwd2), BattVltg > 16/1(BattVltgSwd2)
  BattVltg/1 -> BattVltg <= 16/1(BattVltg), If/1
  If/2 -> BattVltg > 16/Action
  If/1 -> BattVltg <= 16/Action

== system ES259A_BattVltgCorrln/BattVltgCorrln/BattVltgCorrlnPer1/WarmInit or Enable/Instantaneous Correlation/Correlation Check/Copyright1 ==

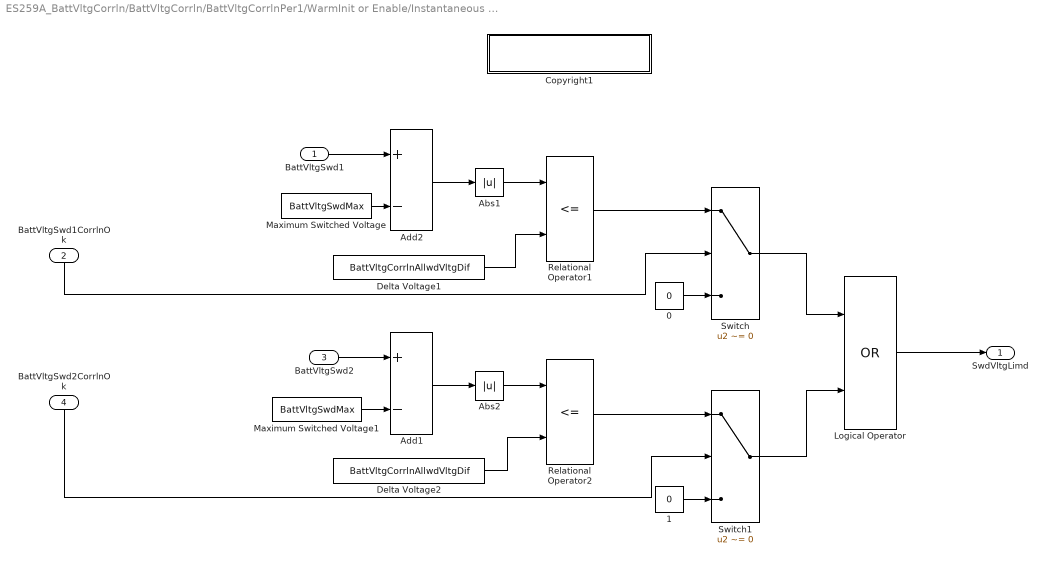
== system ES259A_BattVltgCorrln/BattVltgCorrln/BattVltgCorrlnPer1/WarmInit or Enable/Instantaneous Correlation/Correlation Check/DetermineSwitchedVoltageSaturated ==
  BattVltgSwd1 : Inport
  "BattVltgSwd1CorrlnOk " : Inport  Port=2
  BattVltgSwd2 : Inport  Port=3
  BattVltgSwd2CorrlnOk : Inport  Port=4
  0 : Constant  Value=0  OutDataTypeStr=boolean
  1 : Constant  Value=0  OutDataTypeStr=boolean
  Abs1 : Abs  RequirementInfo={} %GIDa_1bf9d11d_6110_4dd2_bceb_9a35ca0c8b48  OutDataTypeStr=single
  Abs2 : Abs  RequirementInfo={} %GIDa_0b14872c_e8b7_4460_a4e2_3d376d4c36ec  OutDataTypeStr=single
  Add1 : Sum  RequirementInfo={} %GIDa_8493384b_8551_4cb1_988e_f3fc82b6933a  Inputs=+-  AccumDataTypeStr=single
  Add2 : Sum  RequirementInfo={} %GIDa_4e3740af_3723_4e05_9d77_0614bd004ba8  Inputs=+-  AccumDataTypeStr=single
  Copyright1 : Subsystem  Description=|  mask(Copyright Information){none=on}
      | Copyright info block.                                               
      |                                                                     
      | Place copyright information at the top of every subsystem in design.
      mask prompts: none "No parameters"
      mask help: Place copyright information at the top of every subsystem in design.
      mask Display:
      | NxtrConf = 'Nexteer Confidential';
      | 
      | sys = bdroot; %handle for the current model ("system")
      | first = get_param(sys,'Created');
      | if(isempty(first))
      |     first = datestr(now,'yyyy');
      | else
      |     first = first(end-3:end);  %year is last four digits
      | end
      | 
      | last = get_param(sys,'LastModifiedDate');
      | if isempty(last)
      |     last = datestr(now,'yyyy');
      | else
      |     last = last(end-3:end);
      | end
      | 
      | if strcmp(first,last)
      |     fprintf('%s\nCopyright  %s Nexteer',NxtrConf,first);
      | else
      |     fprintf('%s\n%s%s-%s Nexteer',NxtrConf,char(169),first,last);
      | end
  Delta Voltage1 : Constant  Value=BattVltgCorrlnAllwdVltgDif
  Delta Voltage2 : Constant  Value=BattVltgCorrlnAllwdVltgDif
  Logical Operator : Logic  Operator=OR  AllPortsSameDT=off  OutDataTypeStr=boolean
  Maximum Switched Voltage : Constant  Value=BattVltgSwdMax
  Maximum Switched Voltage1 : Constant  Value=BattVltgSwdMax
  Relational Operator1 : RelationalOperator  RequirementInfo={} %GIDa_39795206_589e_4ed2_b3c5_6f8b5b6d689f  Operator=<=  OutDataTypeStr=boolean
  Relational Operator2 : RelationalOperator  RequirementInfo={} %GIDa_e4dc24af_46d8_467a_9001_5b7d25ef6abb  Operator=<=  OutDataTypeStr=boolean
  Switch : Switch  Criteria=u2 ~= 0
  Switch1 : Switch  Criteria=u2 ~= 0
  SwdVltgLimd : Outport
  wires:
  BattVltgSwd2CorrlnOk/1 -> Switch1/2
  "BattVltgSwd1CorrlnOk "/1 -> Switch/2
  Logical Operator/1 -> SwdVltgLimd/1
  Switch1/1 -> Logical Operator/2
  Switch/1 -> Logical Operator/1
  Delta Voltage2/1 -> Relational Operator2/2
  Delta Voltage1/1 -> Relational Operator1/2
  BattVltgSwd2/1 -> Add1/1
  BattVltgSwd1/1 -> Add2/1
  1/1 -> Switch1/3
  Relational Operator2/1 -> Switch1/1
  Abs2/1 -> Relational Operator2/1
  Maximum Switched Voltage1/1 -> Add1/2
  Add1/1 -> Abs2/1
  0/1 -> Switch/3
  Relational Operator1/1 -> Switch/1
  Abs1/1 -> Relational Operator1/1
  Maximum Switched Voltage/1 -> Add2/2
  Add2/1 -> Abs1/1
